simulink model "SingleTrack_RTW"  (Simulink 10.1)
settings: Solver=ode1  StartTime=0.0  StopTime=inf  FixedStep=0.001  RelTol=1e-3
PreLoadFcn:
  | vehicle = 'Car'; if ~length(which('cmcmd')), cmenv; end
  | SingleTrack_RTW_bus
  | SingleTrack_RTW_params
InitFcn:
  | vehicle = 'Car'; if ~length(which('cmcmd')), cmenv; end
  | SingleTrack_RTW_bus
undefined symbols (not defined in the file or in its folder): Car_Bdy1_mass, Car_Steering_i, Car_Whl_Radius, Car_WhlBaseF, Car_WhlBaseR, mEngineMax, PT_DL_iDiff, PT_GearBox_iForwardGears
libraries: CarMaker4SL x7
(part 2 of 3)

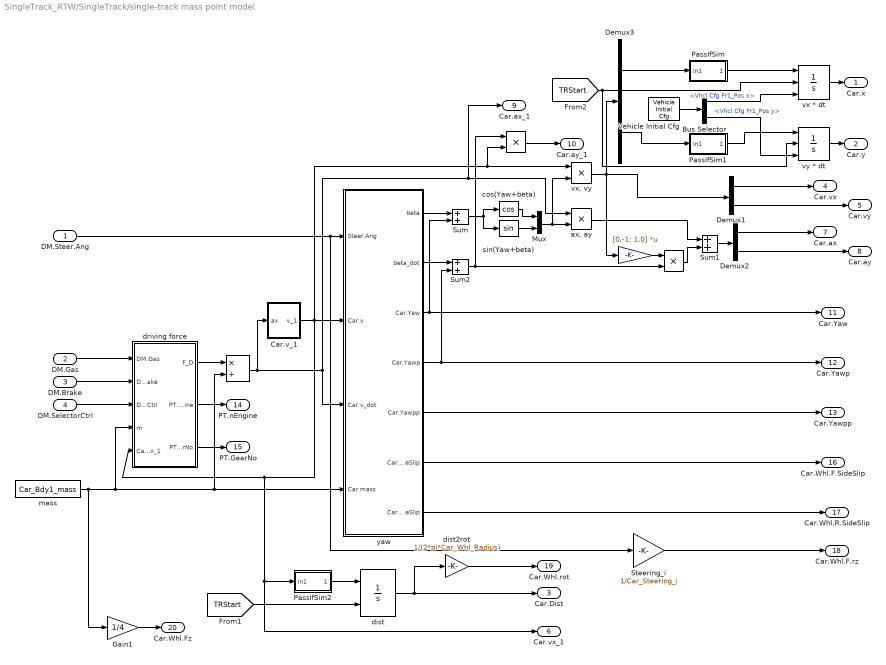
== system SingleTrack_RTW/SingleTrack/single-track mass point model ==
  DM.Steer.Ang : Inport
  DM.Gas : Inport  Port=2
  DM.Brake : Inport  Port=3
  DM.SelectorCtrl : Inport  Port=4
  " " : Gain  Gain=[0,-1; 1,0]  Multiplication=Matrix(K*u)  SaturateOnIntegerOverflow=on  OutDataTypeStr=Inherit: Same as input  ParamDataTypeStr=Inherit: Same as input
  "   " : Product  InputSameDT=on  SaturateOnIntegerOverflow=on  OutDataTypeStr=Inherit: Same as first input
  "     " : Product  InputSameDT=on  SaturateOnIntegerOverflow=on  OutDataTypeStr=Inherit: Same as first input
  "      " : Product  Inputs=*/  InputSameDT=on  SaturateOnIntegerOverflow=on  OutDataTypeStr=Inherit: Same as first input
  Bus Selector : BusSelector  OutputSignals=Vhcl Cfg Fr1_Pos x,Vhcl Cfg Fr1_Pos y
  Car.v_1 : Subsystem
  Demux1 : Demux  Outputs=2
      settings: DisplayOption=none
  Demux2 : Demux  Outputs=2
      settings: DisplayOption=none
  Demux3 : Demux  Outputs=2
      settings: DisplayOption=none
  Gain1 : Gain  Gain=1/4
  Mux : Mux  Inputs=2
  PassIfSim : Subsystem
  PassIfSim1 : Subsystem
  PassIfSim2 : Subsystem
  "Steering_i " : Gain  Gain=1/Car_Steering_i  SaturateOnIntegerOverflow=on  OutDataTypeStr=Inherit: Same as input  ParamDataTypeStr=Inherit: Same as input
  Sum : Sum  InputSameDT=on  SaturateOnIntegerOverflow=on  OutDataTypeStr=Inherit: Same as first input
  Sum1 : Sum  InputSameDT=on  SaturateOnIntegerOverflow=on  OutDataTypeStr=Inherit: Same as first input
  Sum2 : Sum  InputSameDT=on  SaturateOnIntegerOverflow=on  OutDataTypeStr=Inherit: Same as first input
  Vehicle Initial Cfg : CarMaker4SL/Vehicle Initial Cfg
      settings: SourceProductName=CarMaker4SL
  "ax, ay" : Product  InputSameDT=on  SaturateOnIntegerOverflow=on  OutDataTypeStr=Inherit: Same as first input
  cos(Yaw+beta) : Trigonometry  Operator=cos
  dist : Integrator  ExternalReset=level
  dist2rot : Gain  Gain=1/(2*pi*Car_Whl_Radius)  SaturateOnIntegerOverflow=on  OutDataTypeStr=Inherit: Same as input  ParamDataTypeStr=Inherit: Same as input
  driving force : Subsystem
  mass : Constant  Value=Car_Bdy1_mass
  sin(Yaw+beta) : Trigonometry
  vx * dt : Integrator  ExternalReset=level  InitialConditionSource=external  InitialCondition=[0,0]
  "vx, vy" : Product  InputSameDT=on  SaturateOnIntegerOverflow=on  OutDataTypeStr=Inherit: Same as first input
  vy * dt : Integrator  ExternalReset=level  InitialConditionSource=external  InitialCondition=[0,0]
  yaw : Subsystem
  Car.x : Outport  VectorParamsAs1DForOutWhenUnconnected=off
  Car.y : Outport  Port=2  VectorParamsAs1DForOutWhenUnconnected=off
  Car.Dist : Outport  Port=3  VectorParamsAs1DForOutWhenUnconnected=off
  Car.vx : Outport  Port=4  VectorParamsAs1DForOutWhenUnconnected=off
  Car.vy : Outport  Port=5  VectorParamsAs1DForOutWhenUnconnected=off
  Car.vx_1 : Outport  Port=6  VectorParamsAs1DForOutWhenUnconnected=off
  Car.ax : Outport  Port=7  VectorParamsAs1DForOutWhenUnconnected=off
  Car.ay : Outport  Port=8  VectorParamsAs1DForOutWhenUnconnected=off
  Car.ax_1 : Outport  Port=9  VectorParamsAs1DForOutWhenUnconnected=off
  Car.ay_1 : Outport  Port=10  VectorParamsAs1DForOutWhenUnconnected=off
  "Car.Yaw " : Outport  Port=11  VectorParamsAs1DForOutWhenUnconnected=off
  Car.Yawp : Outport  Port=12  VectorParamsAs1DForOutWhenUnconnected=off
  Car.Yawpp : Outport  Port=13  VectorParamsAs1DForOutWhenUnconnected=off
  PT.nEngine : Outport  Port=14  VectorParamsAs1DForOutWhenUnconnected=off
  PT.GearNo : Outport  Port=15  VectorParamsAs1DForOutWhenUnconnected=off
  Car.Whl.F.SideSlip : Outport  Port=16  VectorParamsAs1DForOutWhenUnconnected=off
  Car.Whl.R.SideSlip : Outport  Port=17  VectorParamsAs1DForOutWhenUnconnected=off
  Car.Whl.F.rz : Outport  Port=18  VectorParamsAs1DForOutWhenUnconnected=off
  Car.Whl.rot : Outport  Port=19  VectorParamsAs1DForOutWhenUnconnected=off
  Car.Whl.Fz : Outport  Port=20  VectorParamsAs1DForOutWhenUnconnected=off
  wires:
  [TRStart] -> dist/2
  PassIfSim2/1(Out1) -> dist/1
  PassIfSim1/1(Out1) -> vy * dt/1
  Demux3/2 -> PassIfSim1/1(In1)
  PassIfSim/1(Out1) -> vx * dt/1
  Demux3/1 -> PassIfSim/1(In1)
  dist2rot/1 -> Car.Whl.rot/1
  "Steering_i "/1 -> Car.Whl.F.rz/1
  driving force/2(PT.nEngine) -> PT.nEngine/1
  mass/1 -> "      "/2, yaw/4(Car.mass), driving force/4(m), Gain1/1
  Demux1/1 -> Car.vx/1
  dist/1 -> dist2rot/1, Car.Dist/1
  Demux2/2 -> Car.ay/1
  Demux2/1 -> Car.ax/1
  Demux1/2 -> Car.vy/1
  DM.Gas/1 -> driving force/1(DM.Gas)
  DM.Brake/1 -> driving force/2(DM.Brake)
  driving force/1(F_D) -> "      "/1
  "      "/1 -> "ax, ay"/1, Car.ax_1/1, yaw/3(Car.v_dot), Car.v_1/1(ax)
  yaw/7(Car.Whl.SideSlip) -> Car.Whl.R.SideSlip/1
  yaw/6(Car.Whl.F.SideSlip) -> Car.Whl.F.SideSlip/1
  DM.Steer.Ang/1 -> "Steering_i "/1, yaw/1(Steer.Ang)
  "     "/1 -> Car.ay_1/1
  " "/1 -> "   "/1
  Sum2/1 -> "     "/1, "   "/2
  yaw/2(beta_dot) -> Sum2/1
  "ax, ay"/1 -> Sum1/1
  "   "/1 -> Sum1/2
  Sum1/1 -> Demux2/1
  Car.v_1/1(v_1) -> PassIfSim2/1(In1), Car.vx_1/1, driving force/5(Car.vx_1), "     "/2, "vx, vy"/1, yaw/2(Car.v)
  "vx, vy"/1 -> " "/1, Demux1/1, Demux3/1
  Mux/1 -> "vx, vy"/2, "ax, ay"/2
  yaw/4(Car.Yawp) -> Sum2/2, Car.Yawp/1
  yaw/5(Car.Yawpp) -> Car.Yawpp/1
  Sum/1 -> sin(Yaw+beta)/1, cos(Yaw+beta)/1
  sin(Yaw+beta)/1 -> Mux/2
  cos(Yaw+beta)/1 -> Mux/1
  yaw/3(Car.Yaw) -> "Car.Yaw "/1, Sum/2
  yaw/1(beta) -> Sum/1
  [TRStart] -> vx * dt/2, vy * dt/2
  vy * dt/1 -> Car.y/1
  vx * dt/1 -> Car.x/1
  Vehicle Initial Cfg/1 -> Bus Selector/1
  Bus Selector/2 -> vy * dt/3  "<Vhcl Cfg Fr1_Pos y>"
  Bus Selector/1 -> vx * dt/3  "<Vhcl Cfg Fr1_Pos x>"
  Gain1/1 -> Car.Whl.Fz/1
  driving force/3(PT.GearNo) -> PT.GearNo/1
  DM.SelectorCtrl/1 -> driving force/3(DM.SelectorCtrl)

== system SingleTrack_RTW/SingleTrack_In/CreateBus Vhcl.Misc ==
  In1 : Inport
  Bus Creator5 : BusCreator  Inputs=11
  Demux5 : Demux  Outputs=11
      settings: DisplayOption=none
  Out1 : Outport  VectorParamsAs1DForOutWhenUnconnected=off
  wires:
  Demux5/1 -> Bus Creator5/1  "Vhcl Trq_DL2Bdy1 x"
  Demux5/2 -> Bus Creator5/2  "Vhcl Trq_DL2Bdy1 y"
  Bus Creator5/1 -> Out1/1
  In1/1 -> Demux5/1
  Demux5/3 -> Bus Creator5/3  "Vhcl Trq_DL2Bdy1 z"
  Demux5/4 -> Bus Creator5/4  "Vhcl TrqDL2Bdy1B x"
  Demux5/5 -> Bus Creator5/5  "Vhcl TrqDL2Bdy1B y"
  Demux5/6 -> Bus Creator5/6  "Vhcl TrqDL2Bdy1B z"
  Demux5/7 -> Bus Creator5/7  "Vhcl DL2BdyEng x"
  Demux5/8 -> Bus Creator5/8  "Vhcl DL2BdyEng y"
  Demux5/9 -> Bus Creator5/9  "Vhcl Wind_vel_0 x"
  Demux5/10 -> Bus Creator5/10  "Vhcl Wind_vel_0 y"
  Demux5/11 -> Bus Creator5/11  "Vhcl Wind_vel_0 z"

== system SingleTrack_RTW/SingleTrack_In/CreateBus Vhcl.PT ==
  In1 : Inport
  Bus Creator3 : BusCreator  Inputs=6
  Demux3 : Demux  Outputs=6
      settings: DisplayOption=none
  Out1 : Outport  VectorParamsAs1DForOutWhenUnconnected=off
  wires:
  Demux3/6 -> Bus Creator3/6  "VhclCtrl Gas"
  Demux3/5 -> Bus Creator3/5  "VhclCtrl Clutch"
  Demux3/1 -> Bus Creator3/1  "VhclCtrl Key"
  Demux3/2 -> Bus Creator3/2  "VhclCtrl SST"
  Demux3/3 -> Bus Creator3/3  "VhclCtrl SelectorCtrl"
  Demux3/4 -> Bus Creator3/4  "VhclCtrl GearNo"
  Bus Creator3/1 -> Out1/1
  In1/1 -> Demux3/1

== system SingleTrack_RTW/SingleTrack_In/CreateBus Vhcl.Wheel.In ==
  In1 : Inport
  Bus Creator1 : BusCreator  Inputs=12
  Demux1 : Demux  Outputs=12
      settings: DisplayOption=none
  Out1 : Outport  VectorParamsAs1DForOutWhenUnconnected=off
  wires:
  Demux1/1 -> Bus Creator1/1  "Vhcl Wheel FL Trq_B2WC"
  Demux1/2 -> Bus Creator1/2  "Vhcl Wheel FL Trq_DL2WC"
  Bus Creator1/1 -> Out1/1
  In1/1 -> Demux1/1
  Demux1/3 -> Bus Creator1/3  "Vhcl Wheel FL rotv"
  Demux1/4 -> Bus Creator1/4  "Vhcl Wheel FR Trq_B2WC"
  Demux1/5 -> Bus Creator1/5  "Vhcl Wheel FR Trq_DL2WC"
  Demux1/6 -> Bus Creator1/6  "Vhcl Wheel FR rotv"
  Demux1/7 -> Bus Creator1/7  "Vhcl Wheel RL Trq_B2WC"
  Demux1/8 -> Bus Creator1/8  "Vhcl Wheel RL Trq_DL2WC"
  Demux1/9 -> Bus Creator1/9  "Vhcl Wheel RL rotv"
  Demux1/10 -> Bus Creator1/10  "Vhcl Wheel RR Trq_B2WC"
  Demux1/11 -> Bus Creator1/11  "Vhcl Wheel RR Trq_DL2WC"
  Demux1/12 -> Bus Creator1/12  "Vhcl Wheel RR rotv"

== system SingleTrack_RTW/SingleTrack_In/CreateBus VhclCtrl.Brake ==
  In1 : Inport
  Bus Creator2 : BusCreator  Inputs=2
  Demux2 : Demux  Outputs=2
      settings: DisplayOption=none
  Out1 : Outport  VectorParamsAs1DForOutWhenUnconnected=off
  wires:
  In1/1 -> Demux2/1
  Bus Creator2/1 -> Out1/1
  Demux2/1 -> Bus Creator2/1  "VhclCtrl Brake"
  Demux2/2 -> Bus Creator2/2  "VhclCtrl BrakePark"

== system SingleTrack_RTW/SingleTrack_In/CreateBus VhclCtrl.Steering ==
  In1 : Inport
  Bus Creator : BusCreator  Inputs=5
  Demux : Demux  Outputs=5
      settings: DisplayOption=none
  Out1 : Outport  VectorParamsAs1DForOutWhenUnconnected=off
  wires:
  Demux/4 -> Bus Creator/4  "VhclCtrl Steering Trq"
  Demux/2 -> Bus Creator/2  "VhclCtrl Steering AngVel"
  Demux/3 -> Bus Creator/3  "VhclCtrl Steering AngAcc"
  Demux/5 -> Bus Creator/5  "VhclCtrl Steering ByTrq"
  Demux/1 -> Bus Creator/1  "VhclCtrl Steering Ang"
  Bus Creator/1 -> Out1/1
  In1/1 -> Demux/1

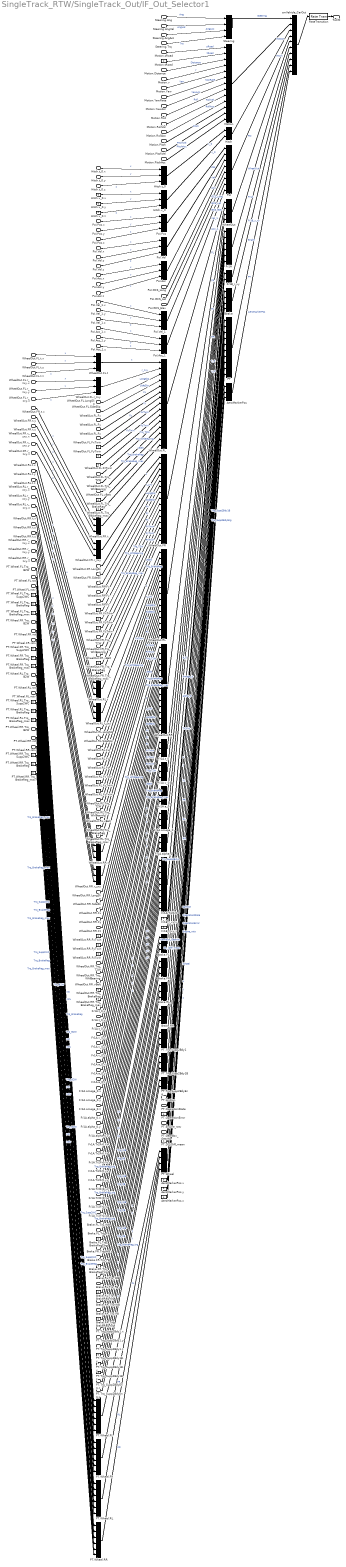
== system SingleTrack_RTW/SingleTrack_Out/IF_Out_Selector1 ==
  Steering.Ang : Inport
  Steering.AngVel : Inport  Port=2
  Steering.AngAcc : Inport  Port=3
  Steering.Trq : Inport  Port=4
  Motion.v : Inport  Port=5
  Motion.Distance : Inport  Port=6
  Motion.sRoad : Inport  Port=7
  Hitch.t_0.x : Inport  Port=8
  Hitch.t_0.y : Inport  Port=9
  Hitch.t_0.z : Inport  Port=10
  Motion.Roll : Inport  Port=11
  Motion.RollVel : Inport  Port=12
  Motion.RollAcc : Inport  Port=13
  Motion.Pitch : Inport  Port=14
  Motion.PitchVel : Inport  Port=15
  Motion.PitchAcc : Inport  Port=16
  Motion.Yaw : Inport  Port=17
  Motion.YawRate : Inport  Port=18
  Motion.YawAcc : Inport  Port=19
  PoI.Pos.x : Inport  Port=20
  PoI.Pos.y : Inport  Port=21
  PoI.Pos.z : Inport  Port=22
  PoI.Vel.x : Inport  Port=23
  PoI.Vel.y : Inport  Port=24
  PoI.Vel.z : Inport  Port=25
  PoI.Acc.x : Inport  Port=26
  PoI.Acc.y : Inport  Port=27
  PoI.Acc.z : Inport  Port=28
  PoI.Vel_1.x : Inport  Port=29
  PoI.Vel_1.y : Inport  Port=30
  PoI.Vel_1.z : Inport  Port=31
  PoI.Acc_1.x : Inport  Port=32
  PoI.Acc_1.y : Inport  Port=33
  PoI.Acc_1.z : Inport  Port=34
  PoI.GCS_Long : Inport  Port=35
  PoI.GCS_Lat : Inport  Port=36
  PoI.GCS_Elev : Inport  Port=37
  WheelOut.FL.t.x : Inport  Port=38
  WheelOut.FL.t.y : Inport  Port=39
  WheelOut.FL.t.z : Inport  Port=40
  WheelOut.FL.r_zxy.x : Inport  Port=41
  WheelOut.FL.r_zxy.y : Inport  Port=42
  WheelOut.FL.r_zxy.z : Inport  Port=43
  WheelOut.FL.Fx : Inport  Port=44
  WheelOut.FL.Fy : Inport  Port=45
  WheelOut.FL.Fz : Inport  Port=46
  WheelOut.FL.vBelt : Inport  Port=47
  WheelOut.FL.LongSlip : Inport  Port=48
  WheelOut.FL.SideSlip : Inport  Port=49
  WheelOut.FL.Trq_T2W : Inport  Port=50
  WheelOut.FL.Trq_WhlBearing : Inport  Port=51
  WheelOut.FR.t.x : Inport  Port=52
  WheelOut.FR.t.y : Inport  Port=53
  WheelOut.FR.t.z : Inport  Port=54
  WheelOut.FR.r_zxy.x : Inport  Port=55
  WheelOut.FR.r_zxy.y : Inport  Port=56
  WheelOut.FR.r_zxy.z : Inport  Port=57
  WheelOut.FR.Fx : Inport  Port=58
  WheelOut.FR.Fy : Inport  Port=59
  WheelOut.FR.Fz : Inport  Port=60
  WheelOut.FR.vBelt : Inport  Port=61
  WheelOut.FR.LongSlip : Inport  Port=62
  WheelOut.FR.SideSlip : Inport  Port=63
  WheelOut.FR.Trq_T2W : Inport  Port=64
  WheelOut.FR.Trq_WhlBearing : Inport  Port=65
  WheelOut.RL.t.x : Inport  Port=66
  WheelOut.RL.t.y : Inport  Port=67
  WheelOut.RL.t.z : Inport  Port=68
  WheelOut.RL.r_zxy.x : Inport  Port=69
  WheelOut.RL.r_zxy.y : Inport  Port=70
  WheelOut.RL.r_zxy.z : Inport  Port=71
  WheelOut.RL.Fx : Inport  Port=72
  WheelOut.RL.Fy : Inport  Port=73
  WheelOut.RL.Fz : Inport  Port=74
  WheelOut.RL.vBelt : Inport  Port=75
  WheelOut.RL.LongSlip : Inport  Port=76
  WheelOut.RL.SideSlip : Inport  Port=77
  WheelOut.RL.Trq_T2W : Inport  Port=78
  WheelOut.RL.Trq_WhlBearing : Inport  Port=79
  WheelOut.RR.t.x : Inport  Port=80
  WheelOut.RR.t.y : Inport  Port=81
  WheelOut.RR.t.z : Inport  Port=82
  WheelOut.RR.r_zxy.x : Inport  Port=83
  WheelOut.RR.r_zxy.y : Inport  Port=84
  WheelOut.RR.r_zxy.z : Inport  Port=85
  WheelOut.RR.Fx : Inport  Port=86
  WheelOut.RR.Fy : Inport  Port=87
  WheelOut.RR.Fz : Inport  Port=88
  WheelOut.RR.vBelt : Inport  Port=89
  WheelOut.RR.LongSlip : Inport  Port=90
  WheelOut.RR.SideSlip : Inport  Port=91
  WheelOut.RR.Trq_T2W : Inport  Port=92
  WheelOut.RR.Trq_WhlBearing : Inport  Port=93
  Fr1A.t_0.x : Inport  Port=94
  Fr1A.t_0.y : Inport  Port=95
  Fr1A.t_0.z : Inport  Port=96
  Fr1A.v_0.x : Inport  Port=97
  Fr1A.v_0.y : Inport  Port=98
  Fr1A.v_0.z : Inport  Port=99
  Fr1A.a_0.x : Inport  Port=100
  Fr1A.a_0.y : Inport  Port=101
  Fr1A.a_0.z : Inport  Port=102
  Fr1A.omega_0.x : Inport  Port=103
  Fr1A.omega_0.y : Inport  Port=104
  Fr1A.omega_0.z : Inport  Port=105
  Fr1A.alpha_0.x : Inport  Port=106
  Fr1A.alpha_0.y : Inport  Port=107
  Fr1A.alpha_0.z : Inport  Port=108
  Fr1A.Tr2Fr0.xx : Inport  Port=109
  Fr1A.Tr2Fr0.xy : Inport  Port=110
  Fr1A.Tr2Fr0.xz : Inport  Port=111
  Fr1A.Tr2Fr0.yx : Inport  Port=112
  Fr1A.Tr2Fr0.yy : Inport  Port=113
  Fr1A.Tr2Fr0.yz : Inport  Port=114
  Fr1A.Tr2Fr0.zx : Inport  Port=115
  Fr1A.Tr2Fr0.zy : Inport  Port=116
  Fr1A.Tr2Fr0.zz : Inport  Port=117
  Brake.FL.Trq_WB : Inport  Port=118
  Brake.FL.Trq_PB : Inport  Port=119
  Brake.FR.Trq_WB : Inport  Port=120
  Brake.FR.Trq_PB : Inport  Port=121
  Brake.RL.Trq_WB : Inport  Port=122
  Brake.RL.Trq_PB : Inport  Port=123
  Brake.RR.Trq_WB : Inport  Port=124
  Brake.RR.Trq_PB : Inport  Port=125
  PT.Trq_Supp2Bdy1.x : Inport  Port=126
  PT.Trq_Supp2Bdy1.y : Inport  Port=127
  PT.Trq_Supp2Bdy1.z : Inport  Port=128
  PT.Trq_Supp2BdyEng.x : Inport  Port=129
  PT.Trq_Supp2BdyEng.y : Inport  Port=130
  PT.Ignition : Inport  Port=131
  PT.Engine_rotv : Inport  Port=132
  PT.GearBox_GearNo : Inport  Port=133
  PT.Wheel.FL.rot : Inport  Port=134
  PT.Wheel.FL.rotv : Inport  Port=135
  PT.Wheel.FL.Trq_B2W : Inport  Port=136
  PT.Wheel.FR.rot : Inport  Port=137
  PT.Wheel.FR.rotv : Inport  Port=138
  PT.Wheel.FR.Trq_B2W : Inport  Port=139
  PT.Wheel.RL.rot : Inport  Port=140
  PT.Wheel.RL.rotv : Inport  Port=141
  PT.Wheel.RL.Trq_B2W : Inport  Port=142
  PT.Wheel.RR.rot : Inport  Port=143
  PT.Wheel.RR.rotv : Inport  Port=144
  PT.Wheel.RR.Trq_B2W : Inport  Port=145
  PT.OperationState : Inport  Port=146
  AeroMarkerPos : BusCreator  Inputs=3
  AeroMarkerPos.x : Constant  Value=0
  AeroMarkerPos.y : Constant  Value=0
  AeroMarkerPos.z : Constant  Value=0
  Brake : BusCreator  Inputs=4
  Brake.FL : BusCreator  Inputs=3
  Brake.FL.Trq_BrakeReg_trg : Constant  Value=0
  Brake.FR : BusCreator  Inputs=3
  Brake.FR.Trq_BrakeReg_trg : Constant  Value=0
  Brake.RL : BusCreator  Inputs=3
  Brake.RL.Trq_BrakeReg_trg : Constant  Value=0
  Brake.RR : BusCreator  Inputs=3
  Brake.RR.Trq_BrakeReg_trg : Constant  Value=0
  Fr1A : BusCreator  Inputs=6
  Fr1A.Tr2Fr0 : BusCreator  Inputs=9
  Fr1A.a_0 : BusCreator  Inputs=3
  Fr1A.alpha_0 : BusCreator  Inputs=3
  Fr1A.omega_0 : BusCreator  Inputs=3
  Fr1A.t_0 : BusCreator  Inputs=3
  Fr1A.v_0 : BusCreator  Inputs=3
  Fr1B_r_xy : BusCreator  Inputs=2
  Fr1B_r_xy.x : Constant  Value=0
  Fr1B_r_xy.y : Constant  Value=0
  Hitch : BusCreator  Inputs=2
  Hitch.t_0 : BusCreator  Inputs=3
  Hitch.v_0 : BusCreator  Inputs=3
  Hitch.v_0.x : Constant  Value=0
  Hitch.v_0.y : Constant  Value=0
  Hitch.v_0.z : Constant  Value=0
  Motion : BusCreator  Inputs=13
  Motion.tRoad : Constant  Value=0
  PT : BusCreator  Inputs=10
  PT.DL_iDiff_mean : Constant  Value=0
  PT.OperationError : Constant  Value=0
  PT.Trq_Supp2Bdy1 : BusCreator  Inputs=3
  PT.Trq_Supp2Bdy1B : BusCreator  Inputs=3
  PT.Trq_Supp2Bdy1B.x : Constant  Value=0
  PT.Trq_Supp2Bdy1B.y : Constant  Value=0
  PT.Trq_Supp2Bdy1B.z : Constant  Value=0
  PT.Trq_Supp2BdyEng : BusCreator  Inputs=2
  PT.Wheel : BusCreator  Inputs=4
  PT.Wheel.FL : BusCreator  Inputs=6
  PT.Wheel.FL.Trq_BrakeReg : Constant  Value=0
  PT.Wheel.FL.Trq_BrakeReg_max : Constant  Value=0
  PT.Wheel.FL.Trq_Supp2WC : Constant  Value=0
  PT.Wheel.FR : BusCreator  Inputs=6
  PT.Wheel.FR.Trq_BrakeReg : Constant  Value=0
  PT.Wheel.FR.Trq_BrakeReg_max : Constant  Value=0
  PT.Wheel.FR.Trq_Supp2WC : Constant  Value=0
  PT.Wheel.RL : BusCreator  Inputs=6
  PT.Wheel.RL.Trq_BrakeReg : Constant  Value=0
  PT.Wheel.RL.Trq_BrakeReg_max : Constant  Value=0
  PT.Wheel.RL.Trq_Supp2WC : Constant  Value=0
  PT.Wheel.RR : BusCreator  Inputs=6
  PT.Wheel.RR.Trq_BrakeReg : Constant  Value=0
  PT.Wheel.RR.Trq_BrakeReg_max : Constant  Value=0
  PT.Wheel.RR.Trq_Supp2WC : Constant  Value=0
  PoI : BusCreator  Inputs=8
  PoI.Acc : BusCreator  Inputs=3
  PoI.Acc_1 : BusCreator  Inputs=3
  PoI.Pos : BusCreator  Inputs=3
  PoI.Vel : BusCreator  Inputs=3
  PoI.Vel_1 : BusCreator  Inputs=3
  RateTransition : RateTransition  OutPortSampleTime=str2num(get_param(bdroot,'FixedStep'))
  Steering : BusCreator  Inputs=4
  WheelOut : BusCreator  Inputs=4
  WheelOut.FL : BusCreator  Inputs=15
  WheelOut.FL.FxTwin : Constant  Value=0
  WheelOut.FL.FyTwin : Constant  Value=0
  WheelOut.FL.FzTwin : Constant  Value=0
  WheelOut.FL.Trq_BrakeReg : Constant  Value=0
  WheelOut.FL.Trq_BrakeReg_max : Constant  Value=0
  WheelOut.FL.r_zxy : BusCreator  Inputs=3
  WheelOut.FL.t : BusCreator  Inputs=3
  WheelOut.FR : BusCreator  Inputs=15
  WheelOut.FR.FxTwin : Constant  Value=0
  WheelOut.FR.FyTwin : Constant  Value=0
  WheelOut.FR.FzTwin : Constant  Value=0
  WheelOut.FR.Trq_BrakeReg : Constant  Value=0
  WheelOut.FR.Trq_BrakeReg_max : Constant  Value=0
  WheelOut.FR.r_zxy : BusCreator  Inputs=3
  WheelOut.FR.t : BusCreator  Inputs=3
  WheelOut.RL : BusCreator  Inputs=15
  WheelOut.RL.FxTwin : Constant  Value=0
  WheelOut.RL.FyTwin : Constant  Value=0
  WheelOut.RL.FzTwin : Constant  Value=0
  WheelOut.RL.Trq_BrakeReg : Constant  Value=0
  WheelOut.RL.Trq_BrakeReg_max : Constant  Value=0
  WheelOut.RL.r_zxy : BusCreator  Inputs=3
  WheelOut.RL.t : BusCreator  Inputs=3
  WheelOut.RR : BusCreator  Inputs=15
  WheelOut.RR.FxTwin : Constant  Value=0
  WheelOut.RR.FyTwin : Constant  Value=0
  WheelOut.RR.FzTwin : Constant  Value=0
  WheelOut.RR.Trq_BrakeReg : Constant  Value=0
  WheelOut.RR.Trq_BrakeReg_max : Constant  Value=0
  WheelOut.RR.r_zxy : BusCreator  Inputs=3
  WheelOut.RR.t : BusCreator  Inputs=3
  cmVehicle_CarOut : BusCreator  Inputs=10
  ToCM : Outport  VectorParamsAs1DForOutWhenUnconnected=off
  wires:
  RateTransition/1 -> ToCM/1
  cmVehicle_CarOut/1 -> RateTransition/1
  Steering/1 -> cmVehicle_CarOut/1  "Steering"
  Motion/1 -> cmVehicle_CarOut/2  "Motion"
  Motion.tRoad/1 -> Motion/2  "tRoad"
  Hitch/1 -> cmVehicle_CarOut/3  "Hitch"
  Hitch.t_0/1 -> Hitch/1  "t_0"
  Hitch.v_0/1 -> Hitch/2  "v_0"
  Hitch.v_0.x/1 -> Hitch.v_0/1  "x"
  Hitch.v_0.y/1 -> Hitch.v_0/2  "y"
  Hitch.v_0.z/1 -> Hitch.v_0/3  "z"
  PoI/1 -> cmVehicle_CarOut/4  "PoI"
  PoI.Pos/1 -> PoI/1  "Pos"
  PoI.Vel/1 -> PoI/2  "Vel"
  PoI.Acc/1 -> PoI/3  "Acc"
  PoI.Vel_1/1 -> PoI/7  "Vel_1"
  PoI.Acc_1/1 -> PoI/8  "Acc_1"
  WheelOut/1 -> cmVehicle_CarOut/5  "WheelOut"
  WheelOut.FL/1 -> WheelOut/1  "FL"
  WheelOut.FL.t/1 -> WheelOut.FL/1  "t"
  WheelOut.FL.r_zxy/1 -> WheelOut.FL/2  "r_zxy"
  WheelOut.FL.FxTwin/1 -> WheelOut.FL/8  "FxTwin"
  WheelOut.FL.FyTwin/1 -> WheelOut.FL/9  "FyTwin"
  WheelOut.FL.FzTwin/1 -> WheelOut.FL/10  "FzTwin"
  WheelOut.FL.Trq_BrakeReg/1 -> WheelOut.FL/14  "Trq_BrakeReg"
  WheelOut.FL.Trq_BrakeReg_max/1 -> WheelOut.FL/15  "Trq_BrakeReg_max"
  WheelOut.FR/1 -> WheelOut/2  "FR"
  WheelOut.FR.t/1 -> WheelOut.FR/1  "t"
  WheelOut.FR.r_zxy/1 -> WheelOut.FR/2  "r_zxy"
  WheelOut.FR.FxTwin/1 -> WheelOut.FR/8  "FxTwin"
  WheelOut.FR.FyTwin/1 -> WheelOut.FR/9  "FyTwin"
  WheelOut.FR.FzTwin/1 -> WheelOut.FR/10  "FzTwin"
  WheelOut.FR.Trq_BrakeReg/1 -> WheelOut.FR/14  "Trq_BrakeReg"
  WheelOut.FR.Trq_BrakeReg_max/1 -> WheelOut.FR/15  "Trq_BrakeReg_max"
  WheelOut.RL/1 -> WheelOut/3  "RL"
  WheelOut.RL.t/1 -> WheelOut.RL/1  "t"
  WheelOut.RL.r_zxy/1 -> WheelOut.RL/2  "r_zxy"
  WheelOut.RL.FxTwin/1 -> WheelOut.RL/8  "FxTwin"
  WheelOut.RL.FyTwin/1 -> WheelOut.RL/9  "FyTwin"
  WheelOut.RL.FzTwin/1 -> WheelOut.RL/10  "FzTwin"
  WheelOut.RL.Trq_BrakeReg/1 -> WheelOut.RL/14  "Trq_BrakeReg"
  WheelOut.RL.Trq_BrakeReg_max/1 -> WheelOut.RL/15  "Trq_BrakeReg_max"
  WheelOut.RR/1 -> WheelOut/4  "RR"
  WheelOut.RR.t/1 -> WheelOut.RR/1  "t"
  WheelOut.RR.r_zxy/1 -> WheelOut.RR/2  "r_zxy"
  WheelOut.RR.FxTwin/1 -> WheelOut.RR/8  "FxTwin"
  WheelOut.RR.FyTwin/1 -> WheelOut.RR/9  "FyTwin"
  WheelOut.RR.FzTwin/1 -> WheelOut.RR/10  "FzTwin"
  WheelOut.RR.Trq_BrakeReg/1 -> WheelOut.RR/14  "Trq_BrakeReg"
  WheelOut.RR.Trq_BrakeReg_max/1 -> WheelOut.RR/15  "Trq_BrakeReg_max"
  Fr1A/1 -> cmVehicle_CarOut/6  "Fr1A"
  Fr1A.t_0/1 -> Fr1A/1  "t_0"
  Fr1A.v_0/1 -> Fr1A/2  "v_0"
  Fr1A.a_0/1 -> Fr1A/3  "a_0"
  Fr1A.omega_0/1 -> Fr1A/4  "omega_0"
  Fr1A.alpha_0/1 -> Fr1A/5  "alpha_0"
  Fr1A.Tr2Fr0/1 -> Fr1A/6  "Tr2Fr0"
  Fr1B_r_xy/1 -> cmVehicle_CarOut/7  "Fr1B_r_xy"
  Fr1B_r_xy.x/1 -> Fr1B_r_xy/1  "x"
  Fr1B_r_xy.y/1 -> Fr1B_r_xy/2  "y"
  Brake/1 -> cmVehicle_CarOut/8  "Brake"
  Brake.FL/1 -> Brake/1  "FL"
  Brake.FL.Trq_BrakeReg_trg/1 -> Brake.FL/3  "Trq_BrakeReg_trg"
  Brake.FR/1 -> Brake/2  "FR"
  Brake.FR.Trq_BrakeReg_trg/1 -> Brake.FR/3  "Trq_BrakeReg_trg"
  Brake.RL/1 -> Brake/3  "RL"
  Brake.RL.Trq_BrakeReg_trg/1 -> Brake.RL/3  "Trq_BrakeReg_trg"
  Brake.RR/1 -> Brake/4  "RR"
  Brake.RR.Trq_BrakeReg_trg/1 -> Brake.RR/3  "Trq_BrakeReg_trg"
  PT/1 -> cmVehicle_CarOut/9  "PT"
  PT.Trq_Supp2Bdy1/1 -> PT/1  "Trq_Supp2Bdy1"
  PT.Trq_Supp2Bdy1B/1 -> PT/2  "Trq_Supp2Bdy1B"
  PT.Trq_Supp2Bdy1B.x/1 -> PT.Trq_Supp2Bdy1B/1  "x"
  PT.Trq_Supp2Bdy1B.y/1 -> PT.Trq_Supp2Bdy1B/2  "y"
  PT.Trq_Supp2Bdy1B.z/1 -> PT.Trq_Supp2Bdy1B/3  "z"
  PT.Trq_Supp2BdyEng/1 -> PT/3  "Trq_Supp2BdyEng"
  PT.OperationError/1 -> PT/6  "OperationError"
  PT.DL_iDiff_mean/1 -> PT/9  "DL_iDiff_mean"
  PT.Wheel/1 -> PT/10  "Wheel"
  PT.Wheel.FL/1 -> PT.Wheel/1  "FL"
  PT.Wheel.FL.Trq_Supp2WC/1 -> PT.Wheel.FL/4  "Trq_Supp2WC"
  PT.Wheel.FL.Trq_BrakeReg/1 -> PT.Wheel.FL/5  "Trq_BrakeReg"
  PT.Wheel.FL.Trq_BrakeReg_max/1 -> PT.Wheel.FL/6  "Trq_BrakeReg_max"
  PT.Wheel.FR/1 -> PT.Wheel/2  "FR"
  PT.Wheel.FR.Trq_Supp2WC/1 -> PT.Wheel.FR/4  "Trq_Supp2WC"
  PT.Wheel.FR.Trq_BrakeReg/1 -> PT.Wheel.FR/5  "Trq_BrakeReg"
  PT.Wheel.FR.Trq_BrakeReg_max/1 -> PT.Wheel.FR/6  "Trq_BrakeReg_max"
  PT.Wheel.RL/1 -> PT.Wheel/3  "RL"
  PT.Wheel.RL.Trq_Supp2WC/1 -> PT.Wheel.RL/4  "Trq_Supp2WC"
  PT.Wheel.RL.Trq_BrakeReg/1 -> PT.Wheel.RL/5  "Trq_BrakeReg"
  PT.Wheel.RL.Trq_BrakeReg_max/1 -> PT.Wheel.RL/6  "Trq_BrakeReg_max"
  PT.Wheel.RR/1 -> PT.Wheel/4  "RR"
  PT.Wheel.RR.Trq_Supp2WC/1 -> PT.Wheel.RR/4  "Trq_Supp2WC"
  PT.Wheel.RR.Trq_BrakeReg/1 -> PT.Wheel.RR/5  "Trq_BrakeReg"
  PT.Wheel.RR.Trq_BrakeReg_max/1 -> PT.Wheel.RR/6  "Trq_BrakeReg_max"
  AeroMarkerPos/1 -> cmVehicle_CarOut/10  "AeroMarkerPos"
  AeroMarkerPos.x/1 -> AeroMarkerPos/1  "x"
  AeroMarkerPos.y/1 -> AeroMarkerPos/2  "y"
  AeroMarkerPos.z/1 -> AeroMarkerPos/3  "z"
  Steering.Ang/1 -> Steering/1  "Ang"
  Steering.AngVel/1 -> Steering/2  "AngVel"
  Steering.AngAcc/1 -> Steering/3  "AngAcc"
  Steering.Trq/1 -> Steering/4  "Trq"
  Motion.v/1 -> Motion/4  "v"
  Motion.Distance/1 -> Motion/3  "Distance"
  Motion.sRoad/1 -> Motion/1  "sRoad"
  Hitch.t_0.x/1 -> Hitch.t_0/1  "x"
  Hitch.t_0.y/1 -> Hitch.t_0/2  "y"
  Hitch.t_0.z/1 -> Hitch.t_0/3  "z"
  Motion.Roll/1 -> Motion/8  "Roll"
  Motion.RollVel/1 -> Motion/9  "RollVel"
  Motion.RollAcc/1 -> Motion/10  "RollAcc"
  Motion.Pitch/1 -> Motion/11  "Pitch"
  Motion.PitchVel/1 -> Motion/12  "PitchVel"
  Motion.PitchAcc/1 -> Motion/13  "PitchAcc"
  Motion.Yaw/1 -> Motion/5  "Yaw"
  Motion.YawRate/1 -> Motion/6  "YawRate"
  Motion.YawAcc/1 -> Motion/7  "YawAcc"
  PoI.Pos.x/1 -> PoI.Pos/1  "x"
  PoI.Pos.y/1 -> PoI.Pos/2  "y"
  PoI.Pos.z/1 -> PoI.Pos/3  "z"
  PoI.Vel.x/1 -> PoI.Vel/1  "x"
  PoI.Vel.y/1 -> PoI.Vel/2  "y"
  PoI.Vel.z/1 -> PoI.Vel/3  "z"
  PoI.Acc.x/1 -> PoI.Acc/1  "x"
  PoI.Acc.y/1 -> PoI.Acc/2  "y"
  PoI.Acc.z/1 -> PoI.Acc/3  "z"
  PoI.Vel_1.x/1 -> PoI.Vel_1/1  "x"
  PoI.Vel_1.y/1 -> PoI.Vel_1/2  "y"
  PoI.Vel_1.z/1 -> PoI.Vel_1/3  "z"
  PoI.Acc_1.x/1 -> PoI.Acc_1/1  "x"
  PoI.Acc_1.y/1 -> PoI.Acc_1/2  "y"
  PoI.Acc_1.z/1 -> PoI.Acc_1/3  "z"
  PoI.GCS_Long/1 -> PoI/4  "GCS_Long"
  PoI.GCS_Lat/1 -> PoI/5  "GCS_Lat"
  PoI.GCS_Elev/1 -> PoI/6  "GCS_Elev"
  WheelOut.FL.t.x/1 -> WheelOut.FL.t/1  "x"
  WheelOut.FL.t.y/1 -> WheelOut.FL.t/2  "y"
  WheelOut.FL.t.z/1 -> WheelOut.FL.t/3  "z"
  WheelOut.FL.r_zxy.x/1 -> WheelOut.FL.r_zxy/1  "x"
  WheelOut.FL.r_zxy.y/1 -> WheelOut.FL.r_zxy/2  "y"
  WheelOut.FL.r_zxy.z/1 -> WheelOut.FL.r_zxy/3  "z"
  WheelOut.FL.Fx/1 -> WheelOut.FL/5  "Fx"
  WheelOut.FL.Fy/1 -> WheelOut.FL/6  "Fy"
  WheelOut.FL.Fz/1 -> WheelOut.FL/7  "Fz"
  WheelOut.FL.vBelt/1 -> WheelOut.FL/13  "vBelt"
  WheelOut.FL.LongSlip/1 -> WheelOut.FL/3  "LongSlip"
  WheelOut.FL.SideSlip/1 -> WheelOut.FL/4  "SideSlip"
  WheelOut.FL.Trq_T2W/1 -> WheelOut.FL/11  "Trq_T2W"
  WheelOut.FL.Trq_WhlBearing/1 -> WheelOut.FL/12  "Trq_WhlBearing"
  WheelOut.FR.t.x/1 -> WheelOut.FR.t/1  "x"
  WheelOut.FR.t.y/1 -> WheelOut.FR.t/2  "y"
  WheelOut.FR.t.z/1 -> WheelOut.FR.t/3  "z"
  WheelOut.FR.r_zxy.x/1 -> WheelOut.FR.r_zxy/1  "x"
  WheelOut.FR.r_zxy.y/1 -> WheelOut.FR.r_zxy/2  "y"
  WheelOut.FR.r_zxy.z/1 -> WheelOut.FR.r_zxy/3  "z"
  WheelOut.FR.Fx/1 -> WheelOut.FR/5  "Fx"
  WheelOut.FR.Fy/1 -> WheelOut.FR/6  "Fy"
  WheelOut.FR.Fz/1 -> WheelOut.FR/7  "Fz"
  WheelOut.FR.vBelt/1 -> WheelOut.FR/13  "vBelt"
  WheelOut.RL.LongSlip/1 -> WheelOut.RL/3  "LongSlip"
  WheelOut.RL.SideSlip/1 -> WheelOut.RL/4  "SideSlip"
  WheelOut.RL.Trq_T2W/1 -> WheelOut.RL/11  "Trq_T2W"
  WheelOut.RL.Trq_WhlBearing/1 -> WheelOut.RL/12  "Trq_WhlBearing"
  WheelOut.FR.LongSlip/1 -> WheelOut.FR/3  "LongSlip"
  WheelOut.FR.SideSlip/1 -> WheelOut.FR/4  "SideSlip"
  WheelOut.FR.Trq_T2W/1 -> WheelOut.FR/11  "Trq_T2W"
  WheelOut.FR.Trq_WhlBearing/1 -> WheelOut.FR/12  "Trq_WhlBearing"
  WheelOut.RL.t.x/1 -> WheelOut.RL.t/1  "x"
  WheelOut.RL.t.y/1 -> WheelOut.RL.t/2  "y"
  WheelOut.RL.t.z/1 -> WheelOut.RL.t/3  "z"
  WheelOut.RL.r_zxy.x/1 -> WheelOut.RL.r_zxy/1  "x"
  WheelOut.RL.r_zxy.y/1 -> WheelOut.RL.r_zxy/2  "y"
  WheelOut.RL.r_zxy.z/1 -> WheelOut.RL.r_zxy/3  "z"
  WheelOut.RL.Fx/1 -> WheelOut.RL/5  "Fx"
  WheelOut.RL.Fy/1 -> WheelOut.RL/6  "Fy"
  WheelOut.RL.Fz/1 -> WheelOut.RL/7  "Fz"
  WheelOut.RL.vBelt/1 -> WheelOut.RL/13  "vBelt"
  WheelOut.RR.t.x/1 -> WheelOut.RR.t/1  "x"
  WheelOut.RR.t.y/1 -> WheelOut.RR.t/2  "y"
  WheelOut.RR.t.z/1 -> WheelOut.RR.t/3  "z"
  WheelOut.RR.r_zxy.x/1 -> WheelOut.RR.r_zxy/1  "x"
  WheelOut.RR.r_zxy.y/1 -> WheelOut.RR.r_zxy/2  "y"
  WheelOut.RR.r_zxy.z/1 -> WheelOut.RR.r_zxy/3  "z"
  WheelOut.RR.Fx/1 -> WheelOut.RR/5  "Fx"
  WheelOut.RR.Fy/1 -> WheelOut.RR/6  "Fy"
  WheelOut.RR.Fz/1 -> WheelOut.RR/7  "Fz"
  WheelOut.RR.vBelt/1 -> WheelOut.RR/13  "vBelt"
  WheelOut.RR.LongSlip/1 -> WheelOut.RR/3  "LongSlip"
  WheelOut.RR.SideSlip/1 -> WheelOut.RR/4  "SideSlip"
  WheelOut.RR.Trq_T2W/1 -> WheelOut.RR/11  "Trq_T2W"
  WheelOut.RR.Trq_WhlBearing/1 -> WheelOut.RR/12  "Trq_WhlBearing"
  Fr1A.t_0.x/1 -> Fr1A.t_0/1  "x"
  Fr1A.t_0.y/1 -> Fr1A.t_0/2  "y"
  Fr1A.t_0.z/1 -> Fr1A.t_0/3  "z"
  Fr1A.v_0.x/1 -> Fr1A.v_0/1  "x"
  Fr1A.v_0.y/1 -> Fr1A.v_0/2  "y"
  Fr1A.v_0.z/1 -> Fr1A.v_0/3  "z"
  Fr1A.a_0.x/1 -> Fr1A.a_0/1  "x"
  Fr1A.a_0.y/1 -> Fr1A.a_0/2  "y"
  Fr1A.a_0.z/1 -> Fr1A.a_0/3  "z"
  Fr1A.omega_0.x/1 -> Fr1A.omega_0/1  "x"
  Fr1A.omega_0.y/1 -> Fr1A.omega_0/2  "y"
  Fr1A.omega_0.z/1 -> Fr1A.omega_0/3  "z"
  Fr1A.alpha_0.x/1 -> Fr1A.alpha_0/1  "x"
  Fr1A.alpha_0.y/1 -> Fr1A.alpha_0/2  "y"
  Fr1A.alpha_0.z/1 -> Fr1A.alpha_0/3  "z"
  Fr1A.Tr2Fr0.xx/1 -> Fr1A.Tr2Fr0/1  "xx"
  Fr1A.Tr2Fr0.xy/1 -> Fr1A.Tr2Fr0/2  "xy"
  Fr1A.Tr2Fr0.xz/1 -> Fr1A.Tr2Fr0/3  "xz"
  Fr1A.Tr2Fr0.yx/1 -> Fr1A.Tr2Fr0/4  "yx"
  Fr1A.Tr2Fr0.yy/1 -> Fr1A.Tr2Fr0/5  "yy"
  Fr1A.Tr2Fr0.yz/1 -> Fr1A.Tr2Fr0/6  "yz"
  Fr1A.Tr2Fr0.zx/1 -> Fr1A.Tr2Fr0/7  "zx"
  Fr1A.Tr2Fr0.zy/1 -> Fr1A.Tr2Fr0/8  "zy"
  Fr1A.Tr2Fr0.zz/1 -> Fr1A.Tr2Fr0/9  "zz"
  PT.Trq_Supp2Bdy1.x/1 -> PT.Trq_Supp2Bdy1/1  "x"
  PT.Trq_Supp2Bdy1.y/1 -> PT.Trq_Supp2Bdy1/2  "y"
  PT.Trq_Supp2Bdy1.z/1 -> PT.Trq_Supp2Bdy1/3  "z"
  PT.Trq_Supp2BdyEng.x/1 -> PT.Trq_Supp2BdyEng/1  "x"
  PT.Trq_Supp2BdyEng.y/1 -> PT.Trq_Supp2BdyEng/2  "y"
  PT.Ignition/1 -> PT/4  "Ignition"
  PT.Engine_rotv/1 -> PT/7  "Engine_rotv"
  PT.GearBox_GearNo/1 -> PT/8  "GearBox_GearNo"
  PT.Wheel.FL.rot/1 -> PT.Wheel.FL/2  "rot"
  PT.Wheel.FL.rotv/1 -> PT.Wheel.FL/3  "rotv"
  PT.Wheel.FL.Trq_B2W/1 -> PT.Wheel.FL/1  "Trq_B2W"
  PT.Wheel.FR.rot/1 -> PT.Wheel.FR/2  "rot"
  PT.Wheel.FR.rotv/1 -> PT.Wheel.FR/3  "rotv"
  PT.Wheel.FR.Trq_B2W/1 -> PT.Wheel.FR/1  "Trq_B2W"
  PT.Wheel.RL.rot/1 -> PT.Wheel.RL/2  "rot"
  PT.Wheel.RL.rotv/1 -> PT.Wheel.RL/3  "rotv"
  PT.Wheel.RL.Trq_B2W/1 -> PT.Wheel.RL/1  "Trq_B2W"
  PT.Wheel.RR.rot/1 -> PT.Wheel.RR/2  "rot"
  PT.Wheel.RR.rotv/1 -> PT.Wheel.RR/3  "rotv"
  PT.Wheel.RR.Trq_B2W/1 -> PT.Wheel.RR/1  "Trq_B2W"
  Brake.FL.Trq_WB/1 -> Brake.FL/1  "Trq_WB"
  Brake.FL.Trq_PB/1 -> Brake.FL/2  "Trq_PB"
  Brake.FR.Trq_WB/1 -> Brake.FR/1  "Trq_WB"
  Brake.FR.Trq_PB/1 -> Brake.FR/2  "Trq_PB"
  Brake.RL.Trq_WB/1 -> Brake.RL/1  "Trq_WB"
  Brake.RL.Trq_PB/1 -> Brake.RL/2  "Trq_PB"
  Brake.RR.Trq_WB/1 -> Brake.RR/1  "Trq_WB"
  Brake.RR.Trq_PB/1 -> Brake.RR/2  "Trq_PB"
  PT.OperationState/1 -> PT/5  "OperationState"

== system SingleTrack_RTW/SingleTrack_Out/Subsystem ==
  In1 : Inport
  Bus Creator{,1..4} (5 alike) : BusCreator  Inputs=3
  foo_Input_Selector2 : BusSelector  OutputSignals=Vhcl PoI_Pos x,Vhcl PoI_Pos y,Vhcl PoI_Pos z,Vhcl PoI_Vel x,Vhcl PoI_Vel y,Vhcl PoI_Vel z,Vhcl PoI_Acc x,Vhcl PoI_Acc y,Vhcl PoI_Acc z,Vhcl PoI_Vel_1 x,Vhcl PoI_Vel_1 y,Vhcl PoI_Vel_1 z,Vhcl PoI_Acc_1 x,Vhcl PoI_Acc_1 y,Vhcl PoI_Acc_1 z,Vhcl PoI_GCS Long,Vhcl PoI_GCS Lat,Vhcl PoI_GCS Elev
  Out1 : Outport  VectorParamsAs1DForOutWhenUnconnected=off
  Out2 : Outport  Port=2  VectorParamsAs1DForOutWhenUnconnected=off
  Out3 : Outport  Port=3  VectorParamsAs1DForOutWhenUnconnected=off
  Out4 : Outport  Port=4  VectorParamsAs1DForOutWhenUnconnected=off
  Out5 : Outport  Port=5  VectorParamsAs1DForOutWhenUnconnected=off
  Out6 : Outport  Port=6  VectorParamsAs1DForOutWhenUnconnected=off
  Out7 : Outport  Port=7  VectorParamsAs1DForOutWhenUnconnected=off
  Out8 : Outport  Port=8  VectorParamsAs1DForOutWhenUnconnected=off
  wires:
  foo_Input_Selector2/18 -> Out8/1  "<Vhcl PoI_GCS Elev>"
  foo_Input_Selector2/17 -> Out7/1  "<Vhcl PoI_GCS Lat>"
  foo_Input_Selector2/16 -> Out6/1  "<Vhcl PoI_GCS Long>"
  Bus Creator4/1 -> Out5/1
  Bus Creator3/1 -> Out4/1
  In1/1 -> foo_Input_Selector2/1
  Bus Creator2/1 -> Out3/1
  Bus Creator1/1 -> Out2/1
  Bus Creator/1 -> Out1/1
  foo_Input_Selector2/15 -> Bus Creator4/3  "<Vhcl PoI_Acc_1 z>"
  foo_Input_Selector2/14 -> Bus Creator4/2  "<Vhcl PoI_Acc_1 y>"
  foo_Input_Selector2/13 -> Bus Creator4/1  "<Vhcl PoI_Acc_1 x>"
  foo_Input_Selector2/12 -> Bus Creator3/3  "<Vhcl PoI_Vel_1 z>"
  foo_Input_Selector2/11 -> Bus Creator3/2  "<Vhcl PoI_Vel_1 y>"
  foo_Input_Selector2/10 -> Bus Creator3/1  "<Vhcl PoI_Vel_1 x>"
  foo_Input_Selector2/9 -> Bus Creator2/3  "<Vhcl PoI_Acc z>"
  foo_Input_Selector2/8 -> Bus Creator2/2  "<Vhcl PoI_Acc y>"
  foo_Input_Selector2/7 -> Bus Creator2/1  "<Vhcl PoI_Acc x>"
  foo_Input_Selector2/6 -> Bus Creator1/3  "<Vhcl PoI_Vel z>"
  foo_Input_Selector2/5 -> Bus Creator1/2  "<Vhcl PoI_Vel y>"
  foo_Input_Selector2/4 -> Bus Creator1/1  "<Vhcl PoI_Vel x>"
  foo_Input_Selector2/3 -> Bus Creator/3  "<Vhcl PoI_Pos z>"
  foo_Input_Selector2/2 -> Bus Creator/2  "<Vhcl PoI_Pos y>"
  foo_Input_Selector2/1 -> Bus Creator/1  "<Vhcl PoI_Pos x>"

== system SingleTrack_RTW/SingleTrack_Out/Subsystem1 ==
  In1 : Inport
  Bus Creator : BusCreator  Inputs=3
  foo_Input_Selector1 : BusSelector  OutputSignals=Vhcl v,Vhcl Distance,Vhcl sRoad,Vhcl sRoadAero,Vhcl Hitch_Pos x,Vhcl Hitch_Pos y,Vhcl Hitch_Pos z,Vhcl Roll,Vhcl RollVel,Vhcl RollAcc,Vhcl Pitch,Vhcl PitchVel,Vhcl PitchAcc,Vhcl Yaw,Vhcl YawRate,Vhcl YawAcc
  Out1 : Outport  VectorParamsAs1DForOutWhenUnconnected=off
  Out2 : Outport  Port=2  VectorParamsAs1DForOutWhenUnconnected=off
  Out3 : Outport  Port=3  VectorParamsAs1DForOutWhenUnconnected=off
  Out6 : Outport  Port=4  VectorParamsAs1DForOutWhenUnconnected=off
  Out7 : Outport  Port=5  VectorParamsAs1DForOutWhenUnconnected=off
  Out8 : Outport  Port=6  VectorParamsAs1DForOutWhenUnconnected=off
  Out9 : Outport  Port=7  VectorParamsAs1DForOutWhenUnconnected=off
  Out10 : Outport  Port=8  VectorParamsAs1DForOutWhenUnconnected=off
  Out11 : Outport  Port=9  VectorParamsAs1DForOutWhenUnconnected=off
  Out12 : Outport  Port=10  VectorParamsAs1DForOutWhenUnconnected=off
  Out13 : Outport  Port=11  VectorParamsAs1DForOutWhenUnconnected=off
  Out14 : Outport  Port=12  VectorParamsAs1DForOutWhenUnconnected=off
  Out15 : Outport  Port=13  VectorParamsAs1DForOutWhenUnconnected=off
  wires:
  In1/1 -> foo_Input_Selector1/1
  foo_Input_Selector1/16 -> Out15/1  "<Vhcl YawAcc>"
  foo_Input_Selector1/15 -> Out14/1  "<Vhcl YawRate>"
  foo_Input_Selector1/14 -> Out13/1  "<Vhcl Yaw>"
  foo_Input_Selector1/13 -> Out12/1  "<Vhcl PitchAcc>"
  foo_Input_Selector1/12 -> Out11/1  "<Vhcl PitchVel>"
  foo_Input_Selector1/11 -> Out10/1  "<Vhcl Pitch>"
  foo_Input_Selector1/10 -> Out9/1  "<Vhcl RollAcc>"
  foo_Input_Selector1/9 -> Out8/1  "<Vhcl RollVel>"
  foo_Input_Selector1/8 -> Out7/1  "<Vhcl Roll>"
  Bus Creator/1 -> Out6/1
  foo_Input_Selector1/3 -> Out3/1  "<Vhcl sRoad>"
  foo_Input_Selector1/2 -> Out2/1  "<Vhcl Distance>"
  foo_Input_Selector1/1 -> Out1/1  "<Vhcl v>"
  foo_Input_Selector1/7 -> Bus Creator/3  "<Vhcl Hitch_Pos z>"
  foo_Input_Selector1/6 -> Bus Creator/2  "<Vhcl Hitch_Pos y>"
  foo_Input_Selector1/5 -> Bus Creator/1  "<Vhcl Hitch_Pos x>"

== system SingleTrack_RTW/SingleTrack_Out/Subsystem2 ==
  In1 : Inport
  Bus Creator : BusCreator  Inputs=3
  Bus Creator1 : BusCreator  Inputs=3
  foo_Input_Selector3 : BusSelector  OutputSignals=Vhcl Wheel FL t x,Vhcl Wheel FL t y,Vhcl Wheel FL t z,Vhcl Wheel FL r_zxy x,Vhcl Wheel FL r_zxy y,Vhcl Wheel FL r_zxy z,Vhcl Wheel FL Fx,Vhcl Wheel FL Fy,Vhcl Wheel FL Fz,Vhcl Wheel FL vBelt,Vhcl Wheel FL LongSlip,Vhcl Wheel FL SideSlip,Vhcl Wheel FL Trq_T2W,Vhcl Wheel FL Trq_WhlBearing
  Out1 : Outport  VectorParamsAs1DForOutWhenUnconnected=off
  Out2 : Outport  Port=2  VectorParamsAs1DForOutWhenUnconnected=off
  Out3 : Outport  Port=3  VectorParamsAs1DForOutWhenUnconnected=off
  Out4 : Outport  Port=4  VectorParamsAs1DForOutWhenUnconnected=off
  Out5 : Outport  Port=5  VectorParamsAs1DForOutWhenUnconnected=off
  Out6 : Outport  Port=6  VectorParamsAs1DForOutWhenUnconnected=off
  Out7 : Outport  Port=7  VectorParamsAs1DForOutWhenUnconnected=off
  Out8 : Outport  Port=8  VectorParamsAs1DForOutWhenUnconnected=off
  Out9 : Outport  Port=9  VectorParamsAs1DForOutWhenUnconnected=off
  Out10 : Outport  Port=10  VectorParamsAs1DForOutWhenUnconnected=off
  wires:
  foo_Input_Selector3/14 -> Out10/1  "<Vhcl Wheel FL Trq_WhlBearing>"
  foo_Input_Selector3/13 -> Out9/1  "<Vhcl Wheel FL Trq_T2W>"
  foo_Input_Selector3/12 -> Out8/1  "<Vhcl Wheel FL SideSlip>"
  foo_Input_Selector3/11 -> Out7/1  "<Vhcl Wheel FL LongSlip>"
  foo_Input_Selector3/10 -> Out6/1  "<Vhcl Wheel FL vBelt>"
  foo_Input_Selector3/9 -> Out5/1  "<Vhcl Wheel FL Fz>"
  foo_Input_Selector3/8 -> Out4/1  "<Vhcl Wheel FL Fy>"
  In1/1 -> foo_Input_Selector3/1
  foo_Input_Selector3/7 -> Out3/1  "<Vhcl Wheel FL Fx>"
  Bus Creator1/1 -> Out2/1
  Bus Creator/1 -> Out1/1
  foo_Input_Selector3/6 -> Bus Creator1/3  "<Vhcl Wheel FL r_zxy z>"
  foo_Input_Selector3/5 -> Bus Creator1/2  "<Vhcl Wheel FL r_zxy y>"
  foo_Input_Selector3/4 -> Bus Creator1/1  "<Vhcl Wheel FL r_zxy x>"
  foo_Input_Selector3/3 -> Bus Creator/3  "<Vhcl Wheel FL t z>"
  foo_Input_Selector3/2 -> Bus Creator/2  "<Vhcl Wheel FL t y>"
  foo_Input_Selector3/1 -> Bus Creator/1  "<Vhcl Wheel FL t x>"

== system SingleTrack_RTW/SingleTrack_Out/Subsystem3 ==
  In1 : Inport
  Bus Creator : BusCreator  Inputs=3
  Bus Creator1 : BusCreator  Inputs=3
  foo_Input_Selector3 : BusSelector  OutputSignals=Vhcl Wheel FR t x,Vhcl Wheel FR t y,Vhcl Wheel FR t z,Vhcl Wheel FR r_zxy x,Vhcl Wheel FR r_zxy y,Vhcl Wheel FR r_zxy z,Vhcl Wheel FR Fx,Vhcl Wheel FR Fy,Vhcl Wheel FR Fz,Vhcl Wheel FR vBelt,Vhcl Wheel FR LongSlip,Vhcl Wheel FR SideSlip,Vhcl Wheel FR Trq_T2W,Vhcl Wheel FR Trq_WhlBearing
  Out1 : Outport  VectorParamsAs1DForOutWhenUnconnected=off
  Out2 : Outport  Port=2  VectorParamsAs1DForOutWhenUnconnected=off
  Out3 : Outport  Port=3  VectorParamsAs1DForOutWhenUnconnected=off
  Out4 : Outport  Port=4  VectorParamsAs1DForOutWhenUnconnected=off
  Out5 : Outport  Port=5  VectorParamsAs1DForOutWhenUnconnected=off
  Out6 : Outport  Port=6  VectorParamsAs1DForOutWhenUnconnected=off
  Out7 : Outport  Port=7  VectorParamsAs1DForOutWhenUnconnected=off
  Out8 : Outport  Port=8  VectorParamsAs1DForOutWhenUnconnected=off
  Out9 : Outport  Port=9  VectorParamsAs1DForOutWhenUnconnected=off
  Out10 : Outport  Port=10  VectorParamsAs1DForOutWhenUnconnected=off
  wires:
  foo_Input_Selector3/14 -> Out10/1  "<Vhcl Wheel FR Trq_WhlBearing>"
  foo_Input_Selector3/13 -> Out9/1  "<Vhcl Wheel FR Trq_T2W>"
  foo_Input_Selector3/12 -> Out8/1  "<Vhcl Wheel FR SideSlip>"
  foo_Input_Selector3/11 -> Out7/1  "<Vhcl Wheel FR LongSlip>"
  foo_Input_Selector3/10 -> Out6/1  "<Vhcl Wheel FR vBelt>"
  foo_Input_Selector3/9 -> Out5/1  "<Vhcl Wheel FR Fz>"
  foo_Input_Selector3/8 -> Out4/1  "<Vhcl Wheel FR Fy>"
  In1/1 -> foo_Input_Selector3/1
  foo_Input_Selector3/7 -> Out3/1  "<Vhcl Wheel FR Fx>"
  Bus Creator1/1 -> Out2/1
  Bus Creator/1 -> Out1/1
  foo_Input_Selector3/6 -> Bus Creator1/3  "<Vhcl Wheel FR r_zxy z>"
  foo_Input_Selector3/5 -> Bus Creator1/2  "<Vhcl Wheel FR r_zxy y>"
  foo_Input_Selector3/4 -> Bus Creator1/1  "<Vhcl Wheel FR r_zxy x>"
  foo_Input_Selector3/3 -> Bus Creator/3  "<Vhcl Wheel FR t z>"
  foo_Input_Selector3/2 -> Bus Creator/2  "<Vhcl Wheel FR t y>"
  foo_Input_Selector3/1 -> Bus Creator/1  "<Vhcl Wheel FR t x>"

== system SingleTrack_RTW/SingleTrack_Out/Subsystem4 ==
  In1 : Inport
  Bus Creator : BusCreator  Inputs=3
  Bus Creator1 : BusCreator  Inputs=3
  foo_Input_Selector3 : BusSelector  OutputSignals=Vhcl Wheel RL t x,Vhcl Wheel RL t y,Vhcl Wheel RL t z,Vhcl Wheel RL r_zxy x,Vhcl Wheel RL r_zxy y,Vhcl Wheel RL r_zxy z,Vhcl Wheel RL Fx,Vhcl Wheel RL Fy,Vhcl Wheel RL Fz,Vhcl Wheel RL vBelt,Vhcl Wheel RL LongSlip,Vhcl Wheel RL SideSlip,Vhcl Wheel RL Trq_T2W,Vhcl Wheel RL Trq_WhlBearing
  Out1 : Outport  VectorParamsAs1DForOutWhenUnconnected=off
  Out2 : Outport  Port=2  VectorParamsAs1DForOutWhenUnconnected=off
  Out3 : Outport  Port=3  VectorParamsAs1DForOutWhenUnconnected=off
  Out4 : Outport  Port=4  VectorParamsAs1DForOutWhenUnconnected=off
  Out5 : Outport  Port=5  VectorParamsAs1DForOutWhenUnconnected=off
  Out6 : Outport  Port=6  VectorParamsAs1DForOutWhenUnconnected=off
  Out7 : Outport  Port=7  VectorParamsAs1DForOutWhenUnconnected=off
  Out8 : Outport  Port=8  VectorParamsAs1DForOutWhenUnconnected=off
  Out9 : Outport  Port=9  VectorParamsAs1DForOutWhenUnconnected=off
  Out10 : Outport  Port=10  VectorParamsAs1DForOutWhenUnconnected=off
  wires:
  foo_Input_Selector3/14 -> Out10/1  "<Vhcl Wheel RL Trq_WhlBearing>"
  foo_Input_Selector3/13 -> Out9/1  "<Vhcl Wheel RL Trq_T2W>"
  foo_Input_Selector3/12 -> Out8/1  "<Vhcl Wheel RL SideSlip>"
  foo_Input_Selector3/11 -> Out7/1  "<Vhcl Wheel RL LongSlip>"
  foo_Input_Selector3/10 -> Out6/1  "<Vhcl Wheel RL vBelt>"
  foo_Input_Selector3/9 -> Out5/1  "<Vhcl Wheel RL Fz>"
  foo_Input_Selector3/8 -> Out4/1  "<Vhcl Wheel RL Fy>"
  In1/1 -> foo_Input_Selector3/1
  foo_Input_Selector3/7 -> Out3/1  "<Vhcl Wheel RL Fx>"
  Bus Creator1/1 -> Out2/1
  Bus Creator/1 -> Out1/1
  foo_Input_Selector3/6 -> Bus Creator1/3  "<Vhcl Wheel RL r_zxy z>"
  foo_Input_Selector3/5 -> Bus Creator1/2  "<Vhcl Wheel RL r_zxy y>"
  foo_Input_Selector3/4 -> Bus Creator1/1  "<Vhcl Wheel RL r_zxy x>"
  foo_Input_Selector3/3 -> Bus Creator/3  "<Vhcl Wheel RL t z>"
  foo_Input_Selector3/2 -> Bus Creator/2  "<Vhcl Wheel RL t y>"
  foo_Input_Selector3/1 -> Bus Creator/1  "<Vhcl Wheel RL t x>"

== system SingleTrack_RTW/SingleTrack_Out/Subsystem5 ==
  In1 : Inport
  Bus Creator : BusCreator  Inputs=3
  Bus Creator1 : BusCreator  Inputs=3
  foo_Input_Selector3 : BusSelector  OutputSignals=Vhcl Wheel RR t x,Vhcl Wheel RR t y,Vhcl Wheel RR t z,Vhcl Wheel RR r_zxy x,Vhcl Wheel RR r_zxy y,Vhcl Wheel RR r_zxy z,Vhcl Wheel RR Fx,Vhcl Wheel RR Fy,Vhcl Wheel RR Fz,Vhcl Wheel RR vBelt,Vhcl Wheel RR LongSlip,Vhcl Wheel RR SideSlip,Vhcl Wheel RR Trq_T2W,Vhcl Wheel RR Trq_WhlBearing
  Out1 : Outport  VectorParamsAs1DForOutWhenUnconnected=off
  Out2 : Outport  Port=2  VectorParamsAs1DForOutWhenUnconnected=off
  Out3 : Outport  Port=3  VectorParamsAs1DForOutWhenUnconnected=off
  Out4 : Outport  Port=4  VectorParamsAs1DForOutWhenUnconnected=off
  Out5 : Outport  Port=5  VectorParamsAs1DForOutWhenUnconnected=off
  Out6 : Outport  Port=6  VectorParamsAs1DForOutWhenUnconnected=off
  Out7 : Outport  Port=7  VectorParamsAs1DForOutWhenUnconnected=off
  Out8 : Outport  Port=8  VectorParamsAs1DForOutWhenUnconnected=off
  Out9 : Outport  Port=9  VectorParamsAs1DForOutWhenUnconnected=off
  Out10 : Outport  Port=10  VectorParamsAs1DForOutWhenUnconnected=off
  wires:
  foo_Input_Selector3/14 -> Out10/1  "<Vhcl Wheel RR Trq_WhlBearing>"
  foo_Input_Selector3/13 -> Out9/1  "<Vhcl Wheel RR Trq_T2W>"
  foo_Input_Selector3/12 -> Out8/1  "<Vhcl Wheel RR SideSlip>"
  foo_Input_Selector3/11 -> Out7/1  "<Vhcl Wheel RR LongSlip>"
  foo_Input_Selector3/10 -> Out6/1  "<Vhcl Wheel RR vBelt>"
  foo_Input_Selector3/9 -> Out5/1  "<Vhcl Wheel RR Fz>"
  foo_Input_Selector3/8 -> Out4/1  "<Vhcl Wheel RR Fy>"
  In1/1 -> foo_Input_Selector3/1
  foo_Input_Selector3/7 -> Out3/1  "<Vhcl Wheel RR Fx>"
  Bus Creator1/1 -> Out2/1
  Bus Creator/1 -> Out1/1
  foo_Input_Selector3/6 -> Bus Creator1/3  "<Vhcl Wheel RR r_zxy z>"
  foo_Input_Selector3/5 -> Bus Creator1/2  "<Vhcl Wheel RR r_zxy y>"
  foo_Input_Selector3/4 -> Bus Creator1/1  "<Vhcl Wheel RR r_zxy x>"
  foo_Input_Selector3/3 -> Bus Creator/3  "<Vhcl Wheel RR t z>"
  foo_Input_Selector3/2 -> Bus Creator/2  "<Vhcl Wheel RR t y>"
  foo_Input_Selector3/1 -> Bus Creator/1  "<Vhcl Wheel RR t x>"

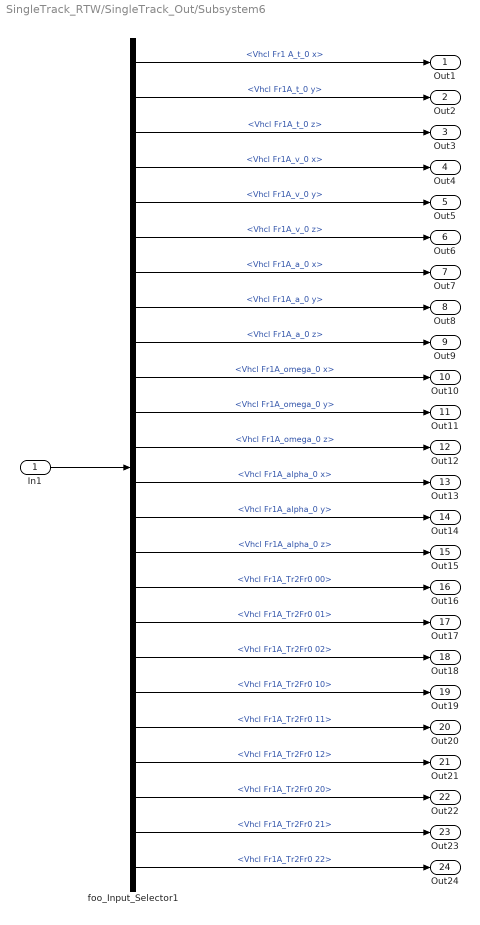
== system SingleTrack_RTW/SingleTrack_Out/Subsystem6 ==
  In1 : Inport
  foo_Input_Selector1 : BusSelector  OutputSignals=Vhcl Fr1 A_t_0 x,Vhcl Fr1A_t_0 y,Vhcl Fr1A_t_0 z,Vhcl Fr1A_v_0 x,Vhcl Fr1A_v_0 y,Vhcl Fr1A_v_0 z,Vhcl Fr1A_a_0 x,Vhcl Fr1A_a_0 y,Vhcl Fr1A_a_0 z,Vhcl Fr1A_omega_0 x,Vhcl Fr1A_omega_0 y,Vhcl Fr1A_omega_0 z,Vhcl Fr1A_alpha_0 x,Vhcl Fr1A_alpha_0 y,Vhcl Fr1A_alpha_0 z,Vhcl Fr1A_Tr2Fr0 00,Vhcl Fr1A_Tr2Fr0 01,Vhcl Fr1A_Tr2Fr0 02,Vhcl Fr1A_Tr2Fr0 10,Vhcl Fr1A_Tr2Fr0 11,Vhcl Fr1A_Tr2Fr0 12,Vhcl Fr1A_Tr2Fr0 20,Vhcl Fr1A_Tr2Fr0 21,Vhcl Fr1A_Tr2Fr0 22
  Out1 : Outport  VectorParamsAs1DForOutWhenUnconnected=off
  Out2 : Outport  Port=2  VectorParamsAs1DForOutWhenUnconnected=off
  Out3 : Outport  Port=3  VectorParamsAs1DForOutWhenUnconnected=off
  Out4 : Outport  Port=4  VectorParamsAs1DForOutWhenUnconnected=off
  Out5 : Outport  Port=5  VectorParamsAs1DForOutWhenUnconnected=off
  Out6 : Outport  Port=6  VectorParamsAs1DForOutWhenUnconnected=off
  Out7 : Outport  Port=7  VectorParamsAs1DForOutWhenUnconnected=off
  Out8 : Outport  Port=8  VectorParamsAs1DForOutWhenUnconnected=off
  Out9 : Outport  Port=9  VectorParamsAs1DForOutWhenUnconnected=off
  Out10 : Outport  Port=10  VectorParamsAs1DForOutWhenUnconnected=off
  Out11 : Outport  Port=11  VectorParamsAs1DForOutWhenUnconnected=off
  Out12 : Outport  Port=12  VectorParamsAs1DForOutWhenUnconnected=off
  Out13 : Outport  Port=13  VectorParamsAs1DForOutWhenUnconnected=off
  Out14 : Outport  Port=14  VectorParamsAs1DForOutWhenUnconnected=off
  Out15 : Outport  Port=15  VectorParamsAs1DForOutWhenUnconnected=off
  Out16 : Outport  Port=16  VectorParamsAs1DForOutWhenUnconnected=off
  Out17 : Outport  Port=17  VectorParamsAs1DForOutWhenUnconnected=off
  Out18 : Outport  Port=18  VectorParamsAs1DForOutWhenUnconnected=off
  Out19 : Outport  Port=19  VectorParamsAs1DForOutWhenUnconnected=off
  Out20 : Outport  Port=20  VectorParamsAs1DForOutWhenUnconnected=off
  Out21 : Outport  Port=21  VectorParamsAs1DForOutWhenUnconnected=off
  Out22 : Outport  Port=22  VectorParamsAs1DForOutWhenUnconnected=off
  Out23 : Outport  Port=23  VectorParamsAs1DForOutWhenUnconnected=off
  Out24 : Outport  Port=24  VectorParamsAs1DForOutWhenUnconnected=off
  wires:
  foo_Input_Selector1/15 -> Out15/1  "<Vhcl Fr1A_alpha_0 z>"
  foo_Input_Selector1/14 -> Out14/1  "<Vhcl Fr1A_alpha_0 y>"
  foo_Input_Selector1/13 -> Out13/1  "<Vhcl Fr1A_alpha_0 x>"
  foo_Input_Selector1/12 -> Out12/1  "<Vhcl Fr1A_omega_0 z>"
  foo_Input_Selector1/11 -> Out11/1  "<Vhcl Fr1A_omega_0 y>"
  foo_Input_Selector1/10 -> Out10/1  "<Vhcl Fr1A_omega_0 x>"
  foo_Input_Selector1/9 -> Out9/1  "<Vhcl Fr1A_a_0 z>"
  foo_Input_Selector1/8 -> Out8/1  "<Vhcl Fr1A_a_0 y>"
  foo_Input_Selector1/7 -> Out7/1  "<Vhcl Fr1A_a_0 x>"
  foo_Input_Selector1/6 -> Out6/1  "<Vhcl Fr1A_v_0 z>"
  foo_Input_Selector1/5 -> Out5/1  "<Vhcl Fr1A_v_0 y>"
  foo_Input_Selector1/4 -> Out4/1  "<Vhcl Fr1A_v_0 x>"
  foo_Input_Selector1/3 -> Out3/1  "<Vhcl Fr1A_t_0 z>"
  foo_Input_Selector1/2 -> Out2/1  "<Vhcl Fr1A_t_0 y>"
  foo_Input_Selector1/1 -> Out1/1  "<Vhcl Fr1 A_t_0 x>"
  In1/1 -> foo_Input_Selector1/1
  foo_Input_Selector1/16 -> Out16/1  "<Vhcl Fr1A_Tr2Fr0 00>"
  foo_Input_Selector1/17 -> Out17/1  "<Vhcl Fr1A_Tr2Fr0 01>"
  foo_Input_Selector1/18 -> Out18/1  "<Vhcl Fr1A_Tr2Fr0 02>"
  foo_Input_Selector1/19 -> Out19/1  "<Vhcl Fr1A_Tr2Fr0 10>"
  foo_Input_Selector1/20 -> Out20/1  "<Vhcl Fr1A_Tr2Fr0 11>"
  foo_Input_Selector1/21 -> Out21/1  "<Vhcl Fr1A_Tr2Fr0 12>"
  foo_Input_Selector1/22 -> Out22/1  "<Vhcl Fr1A_Tr2Fr0 20>"
  foo_Input_Selector1/23 -> Out23/1  "<Vhcl Fr1A_Tr2Fr0 21>"
  foo_Input_Selector1/24 -> Out24/1  "<Vhcl Fr1A_Tr2Fr0 22>"

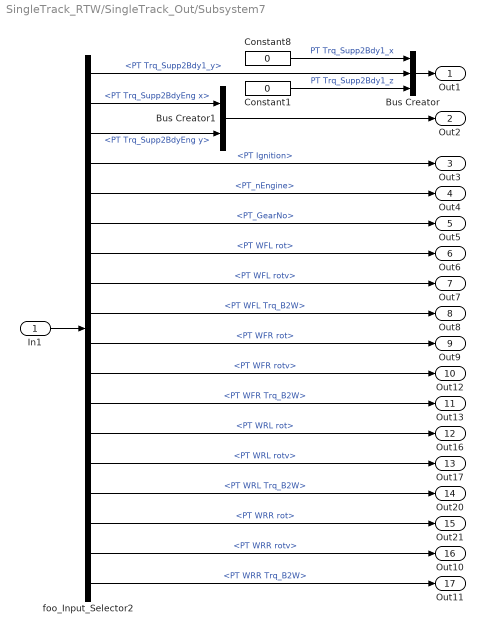
== system SingleTrack_RTW/SingleTrack_Out/Subsystem7 ==
  In1 : Inport
  Bus Creator : BusCreator  Inputs=3
  Bus Creator1 : BusCreator  Inputs=2
  Constant1 : Constant  Value=0
  Constant8 : Constant  Value=0
  foo_Input_Selector2 : BusSelector  OutputSignals=PT Trq_Supp2Bdy1_y,PT Trq_Supp2BdyEng x,PT Trq_Supp2BdyEng y,PT Ignition,PT_nEngine,PT_GearNo,PT WFL rot,PT WFL rotv,PT WFL Trq_B2W,PT WFR rot,PT WFR rotv,PT WFR Trq_B2W,PT WRL rot,PT WRL rotv,PT WRL Trq_B2W,PT WRR rot,PT WRR rotv,PT WRR Trq_B2W
  Out1 : Outport  VectorParamsAs1DForOutWhenUnconnected=off
  Out2 : Outport  Port=2  VectorParamsAs1DForOutWhenUnconnected=off
  Out3 : Outport  Port=3  VectorParamsAs1DForOutWhenUnconnected=off
  Out4 : Outport  Port=4  VectorParamsAs1DForOutWhenUnconnected=off
  Out5 : Outport  Port=5  VectorParamsAs1DForOutWhenUnconnected=off
  Out6 : Outport  Port=6  VectorParamsAs1DForOutWhenUnconnected=off
  Out7 : Outport  Port=7  VectorParamsAs1DForOutWhenUnconnected=off
  Out8 : Outport  Port=8  VectorParamsAs1DForOutWhenUnconnected=off
  Out9 : Outport  Port=9  VectorParamsAs1DForOutWhenUnconnected=off
  Out12 : Outport  Port=10  VectorParamsAs1DForOutWhenUnconnected=off
  Out13 : Outport  Port=11  VectorParamsAs1DForOutWhenUnconnected=off
  Out16 : Outport  Port=12  VectorParamsAs1DForOutWhenUnconnected=off
  Out17 : Outport  Port=13  VectorParamsAs1DForOutWhenUnconnected=off
  Out20 : Outport  Port=14  VectorParamsAs1DForOutWhenUnconnected=off
  Out21 : Outport  Port=15  VectorParamsAs1DForOutWhenUnconnected=off
  Out10 : Outport  Port=16  VectorParamsAs1DForOutWhenUnconnected=off
  Out11 : Outport  Port=17  VectorParamsAs1DForOutWhenUnconnected=off
  wires:
  Bus Creator/1 -> Out1/1
  Constant8/1 -> Bus Creator/1  "PT Trq_Supp2Bdy1_x"
  foo_Input_Selector2/1 -> Bus Creator/2  "<PT Trq_Supp2Bdy1_y>"
  foo_Input_Selector2/2 -> Bus Creator1/1  "<PT Trq_Supp2BdyEng x>"
  foo_Input_Selector2/3 -> Bus Creator1/2  "<PT Trq_Supp2BdyEng y>"
  Bus Creator1/1 -> Out2/1
  foo_Input_Selector2/4 -> Out3/1  "<PT Ignition>"
  foo_Input_Selector2/5 -> Out4/1  "<PT_nEngine>"
  foo_Input_Selector2/6 -> Out5/1  "<PT_GearNo>"
  foo_Input_Selector2/7 -> Out6/1  "<PT WFL rot>"
  foo_Input_Selector2/8 -> Out7/1  "<PT WFL rotv>"
  foo_Input_Selector2/9 -> Out8/1  "<PT WFL Trq_B2W>"
  foo_Input_Selector2/10 -> Out9/1  "<PT WFR rot>"
  Constant1/1 -> Bus Creator/3  "PT Trq_Supp2Bdy1_z"
  In1/1 -> foo_Input_Selector2/1
  foo_Input_Selector2/11 -> Out12/1  "<PT WFR rotv>"
  foo_Input_Selector2/12 -> Out13/1  "<PT WFR Trq_B2W>"
  foo_Input_Selector2/13 -> Out16/1  "<PT WRL rot>"
  foo_Input_Selector2/14 -> Out17/1  "<PT WRL rotv>"
  foo_Input_Selector2/15 -> Out20/1  "<PT WRL Trq_B2W>"
  foo_Input_Selector2/16 -> Out21/1  "<PT WRR rot>"
  foo_Input_Selector2/17 -> Out10/1  "<PT WRR rotv>"
  foo_Input_Selector2/18 -> Out11/1  "<PT WRR Trq_B2W>"
